simulink library "tqd"  (R2021b)
settings: Solver=VariableStepAuto  StartTime=0.0  StopTime=10.0  RelTol=1e-3
undefined symbols (not defined in the file): ATQD_AfterTqMinGain_X_Deg, ATQD_APSCreepBaseTqD_X_kph, ATQD_APSCreepBaseTqD_Y_Deg, ATQD_APSCreepBaseTqR_X_kph, ATQD_APSCreepBaseTqR_Y_Deg, ATQD_APSCreepIterm_X_kph, ATQD_APSCreepIterm_Y_kph, ATQD_APSCreepPterm_X_kph, ATQD_APSCreepPterm_Y_kph, ATQD_APSDecReq_X_kph, ATQD_APSDecReq_Y_mps2, ATQD_APSDecReqCMD_X_kph, ATQD_APSDecReqTs_X_pct, ATQD_APSDecTimeGain_X_Deg, ATQD_APSDecTimeGain_Y_s, ATQD_APSReqLowSpd_X_Deg, ATQD_AutoHoldReleaseBPS_X_Deg, ATQD_AWDLoadTrqnsGain_X_kg, ATQD_AWDLoadTrqnsGain_Y_pct, ATQD_BOSEnBPSPosn_X_kph, ATQD_BOSMap_X_rpm, ATQD_BOSMap_Y_pct, ATQD_CreepBaseTqD_X_kph, ATQD_CreepBaseTqD_Y_Deg, ATQD_CreepBaseTqR_X_kph, ATQD_CreepBaseTqR_Y_Deg, ATQD_CreepBPSDisPosn_X_Deg, ATQD_CreepBPSDisPosnR_X_Deg, ATQD_CreepBPSEnPosn_X_Deg, ATQD_CreepBPSEnPosnR_X_Deg, ATQD_CreepDeltaTq_X_kph, ATQD_CreepIterm_X_kph, ATQD_CreepIterm_Y_kph, ATQD_CreepItermMaxLimit_X_pct, ATQD_CreepPreloadTime_X_kph, ATQD_CreepPreloadTq_X_kph, ATQD_CreepPreloadTq_Y_s, ATQD_CreepProtTq_X_Deg, ATQD_CreepPterm_X_kph, ATQD_CreepPterm_Y_kph, ATQD_CreepRrTqSpRat_X_rpm, ATQD_CreepRrTqSpRat_Y_Nm, ATQD_CreepTargetSpdD_X_pct, ATQD_CreepTargetSpdR_X_pct, ATQD_ECOTqMapD_X_rpm, ATQD_ECOTqMapD_Y_pct, ATQD_EMTqMapD_X_rpm, ATQD_EMTqMapD_Y_pct, ATQD_EOPDTqMapDCon_X_rpm, ATQD_EOPDTqMapDCon_Y_Deg, ATQD_EscapeModePedTq_X_pct, ATQD_EscapeModePedTq_Y_rpm, ATQD_EscapeModePedTqFr_X_pct, ATQD_EscapeModePedTqFr_Y_rpm, ATQD_EstInitVehWeight_X_c, ATQD_FAfterTqCMDGain_X_rpm, ATQD_FAfterTqCMDGain_Y_pct, ATQD_FrLossMAPLowV_X_rpm, ATQD_FrLossMAPLowV_Y_Nm, ATQD_FrMotActReduce_X_rpm ... (+772)
libraries: simulink x211, hcu_lib x179, tqr x3
(part 11 of 28)

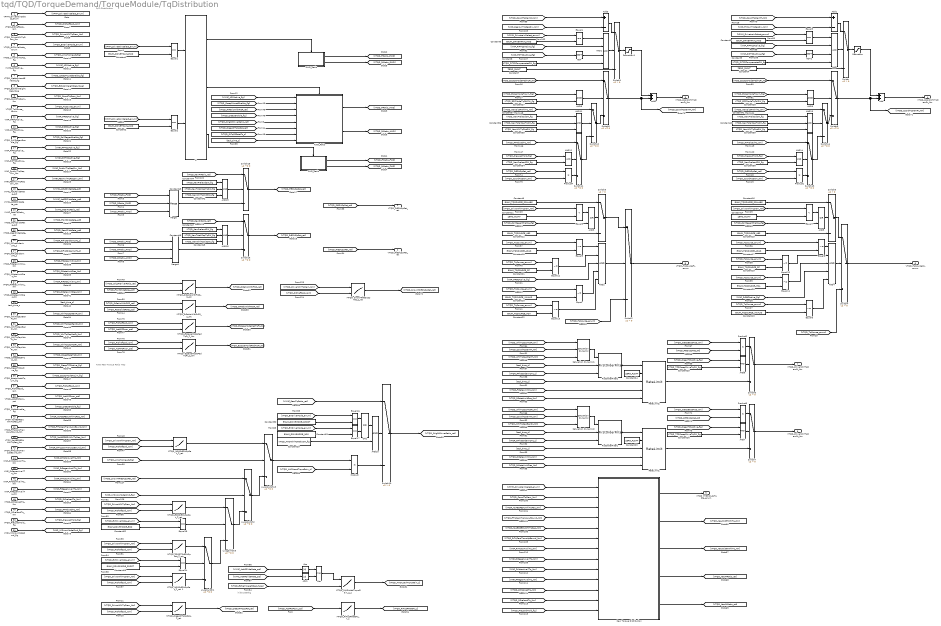
== system tqd/TQD/TorqueDemand/TorqueModule/TqDistribution ==
  note: AWD Rear Torque Ratio Map
  note: Fr/Rr Distribution
  note: initia:2000kg
  VPMM_DrivetrainSelect_enum : Inport
  VTQD_RrShaftSpd_rpm : Inport  Port=2
  VTQD_DriverWhlTqDem_Nm : Inport  Port=3
  VTQD_EVDriveMode_enum : Inport  Port=4
  VTQD_LimpHomeAct_flg : Inport  Port=5
  VVMC_APSActive_flg : Inport  Port=6
  VTQD_CreepPrLoadEnable_flg : Inport  Port=7
  VTQD_EstVehWeightResult_kg : Inport  Port=8
  VTQD_CoordTqDem_Nm : Inport  Port=9
  VTQD_TqSource_enum : Inport  Port=10
  VINP_FrRBCActive_flg : Inport  Port=11
  VINP_RrRBCActive_flg : Inport  Port=12
  VTQD_RollRegenEnable_flg : Inport  Port=13
  VINP_FrPTCSActive_flg : Inport  Port=14
  VINP_RrPTCSActive_flg : Inport  Port=15
  VINP_FrntAxlTrqReqDrv_Nm : Inport  Port=16
  VINP_RearAxlTrqReqDrv_Nm : Inport  Port=17
  VVMC_ActLRSlideRate_pct : Inport  Port=18
  VVMC_ActRRSlideRate_pct : Inport  Port=19
  VVMC_RearTqRatio_rat : Inport  Port=20
  VTQD_FrontSlideRate_pct : Inport  Port=21
  VTQD_RearSlideRate_pct : Inport  Port=22
  VTQR_FrFirstOrderInpTs_c : Inport  Port=23
  VTQR_RrFirstOrderInpTs_c : Inport  Port=24
  VTQR_FrRateLimitInc_Nm : Inport  Port=25
  VTQR_FrRateLimitDec_Nm : Inport  Port=26
  VTQR_RrRateLimitInc_Nm : Inport  Port=27
  VTQR_RrRateLimitDec_Nm : Inport  Port=28
  task_time_s : Inport  Port=29
  VTQD_WhlTqCapGenFr_Nm : Inport  Port=30
  VTQD_WhlTqCapGenRr_Nm : Inport  Port=31
  VTQD_WhlTqCapMotFr_Nm : Inport  Port=32
  VTQD_WhlTqCapMotRr_Nm : Inport  Port=33
  VTQD_CreepBaseTqD_Nm : Inport  Port=34
  VTQD_CreepTCSActive_flg : Inport  Port=35
  VTQD_EscapModeTqLim_flg : Inport  Port=36
  VTQD_FrShaftSpd_rpm : Inport  Port=37
  VTQD_ActAPSPosn_pct : Inport  Port=38
  VTQD_CreepEnable_flg : Inport  Port=39
  VTQR_NoABSFEDUWhlTqReq_Nm : Inport  Port=40
  VTQR_FrTqZeroTransLowBound_Nm : Inport  Port=41
  VTQR_NoABSREDUWhlTqReq_Nm : Inport  Port=42
  VTQR_RrTqZeroTransUpBound_Nm : Inport  Port=43
  VINP_RrMotorAvailTq_Nm : Inport  Port=44
  VINP_RrRegenAvailTq_Nm : Inport  Port=45
  VINP_FrMotorAvailTq_Nm : Inport  Port=46
  VINP_FrRegenAvailTq_Nm : Inport  Port=47
  VTQD_RrPreloadTq_Nm : Inport  Port=48
  VTQD_FrPreloadTq_Nm : Inport  Port=49
  VTQD_PreLoadHold_flg : Inport  Port=50
  VINP_IVISnowModeCmd_flg : Inport  Port=51
  AND : Logic  Inputs=4  AllPortsSameDT=off  OutDataTypeStr=boolean
  AND1 : Logic  Inputs=4  AllPortsSameDT=off  OutDataTypeStr=boolean
  AND{6..10,12,14} (7 alike) : Logic  AllPortsSameDT=off  OutDataTypeStr=boolean
  AND{11,13,15..16} (4 alike) : Logic  Inputs=3  AllPortsSameDT=off  OutDataTypeStr=boolean
  AND2 : Logic  Inputs=5  AllPortsSameDT=off  OutDataTypeStr=boolean
  AND3 : Logic  Operator=OR  AllPortsSameDT=off  OutDataTypeStr=boolean
  AND4 : Logic  Inputs=5  AllPortsSameDT=off  OutDataTypeStr=boolean
  AND5 : Logic  Operator=OR  AllPortsSameDT=off  OutDataTypeStr=boolean
  AWD_Ratio : Subsystem  TreatAsAtomicUnit=on
  Abs : Abs
  Abs1 : Abs
  Add : Sum
  Add1 : Sum  Inputs=+-
  Add2 : Sum
  Add3 : Sum  Inputs=+-
  Constant1 : Constant  Value=ENUM_DRIVETRAIN_RWD  VectorParams1D=off  SampleTime=-1
  Constant10 : Constant  Value=ENUM_TQSOURCE_INVALID  VectorParams1D=off  SampleTime=-1
  Constant{4,7,11,14} (4 alike) : Constant  Value=ZERO_FLOAT  VectorParams1D=off  SampleTime=-1
  Constant12 : Constant  Value=ENUM_TQSOURCE_ABS  VectorParams1D=off  SampleTime=-1
  Constant13 : Constant  Value=ENUM_TQSOURCE_INVALID  VectorParams1D=off  SampleTime=-1
  Constant15 : Constant  Value=ENUM_TQSOURCE_ABS  VectorParams1D=off  SampleTime=-1
  Constant16 : Constant  Value=ENUM_TQSOURCE_ROLLABS  VectorParams1D=off  SampleTime=-1
  Constant17 : Constant  Value=ENUM_TQSOURCE_ADAS  VectorParams1D=off  SampleTime=-1
  Constant18 : Constant  Value=ENUM_TQSOURCE_ADAS  VectorParams1D=off  SampleTime=-1
  Constant19 : Constant  Value=ENUM_TQSOURCE_CC  SampleTime=-1
  Constant2 : Constant  Value=ENUM_DRIVETRAIN_AWD  VectorParams1D=off  SampleTime=-1
  Constant20 : Constant  Value=ENUM_TQSOURCE_MSA  SampleTime=-1
  Constant21 : Constant  Value=ENUM_TQSOURCE_CC  SampleTime=-1
  Constant22 : Constant  Value=ENUM_TQSOURCE_MSA  SampleTime=-1
  Constant23 : Constant  Value=ZERO_FLOAT
  Constant24 : Constant  Value=ZERO_FLOAT
  Constant25 : Constant  Value=KTQD_TCSCreepDriveTqSW_flg  VectorParams1D=off  SampleTime=-1
  Constant26 : Constant  Value=KTQD_TCSCreepDriveTqSW_flg  VectorParams1D=off  SampleTime=-1
  Constant27 : Constant  Value=KTQD_ESCModeTqCtrlSW_flg  VectorParams1D=off  SampleTime=-1
  Constant28 : Constant  Value=KTQD_ESCModeTqCtrlSW_flg  VectorParams1D=off  SampleTime=-1
  Constant29 : Constant  Value=KTQD_AWDWhlTqRatioSW_flg
  Constant3 : Constant  Value=ENUM_DRIVETRAIN_AWD  VectorParams1D=off  SampleTime=-1
  Constant30 : Constant  Value=ENUM_DRIVEMODE_SPORT
  Constant31 : Constant  Value=ENUM_DRIVEMODE_NRM
  Constant32 : Constant  Value=ENUM_DRIVEMODE_ECO
  Constant33 : Constant  Value=ENUM_DRIVEMODE_SPORT
  Constant{34,37..38,41,44,47} (6 alike) : Constant  Value=KTQD_NewPrelaodSW_flg  VectorParams1D=off  SampleTime=-1
  Constant{35,39,42,45} (4 alike) : Constant  Value=KTQD_NewWhlTqDistSW_flg  VectorParams1D=off  SampleTime=-1
  Constant{36,40,43,46} (4 alike) : Constant  Value=KTQD_NewTotalCapTqSW_flg  VectorParams1D=off  SampleTime=-1
  Constant5 : Constant  Value=KTQD_RrTCSCompensateSW_flg  VectorParams1D=off  SampleTime=-1
  Constant6 : Constant  Value=ENUM_DRIVETRAIN_AWD  VectorParams1D=off  SampleTime=-1
  Constant8 : Constant  Value=KTQD_FrTCSCompensateSW_flg  VectorParams1D=off  SampleTime=-1
  Constant9 : Constant  Value=ENUM_TQSOURCE_ROLLABS  VectorParams1D=off  SampleTime=-1
  Equal{,6,8..13} (8 alike) : RelationalOperator  Operator=~=  OutDataTypeStr=boolean  RndMeth=Simplest
  Equal{1..4,14..17} (8 alike) : RelationalOperator  Operator===  OutDataTypeStr=boolean  RndMeth=Simplest
  Equal5 : RelationalOperator  Operator=<  OutDataTypeStr=boolean  RndMeth=Simplest
  Equal7 : RelationalOperator  Operator=<  OutDataTypeStr=boolean  RndMeth=Simplest
  FWD_Ratio : Subsystem  TreatAsAtomicUnit=on
  FirstOrderFilter1 : hcu_lib/Basic_Blocks/FirstOrderFilter
  FirstOrderFilter2 : hcu_lib/Basic_Blocks/FirstOrderFilter
  If : If  NumInputs=2  IfExpression=u1 ~= 0  ElseIfExpressions=u2 ~= 0
  LiuzgSwitch{1..3,13} (4 alike) : Switch  Criteria=u2 ~= 0
      settings: AttributesFormatString=<%<Criteria>>
  MTQD_AWDLoadTrqnsGain_Z_c : Lookup_n-D  BreakpointsForDimension1=ATQD_AWDLoadTrqnsGain_Y_pct  BreakpointsForDimension2=ATQD_AWDLoadTrqnsGain_X_kg  Table=MTQD_AWDLoadTrqnsGain_Z_c  ExtrapMethod=Clip  InternalRulePriority=Speed  RndMeth=Simplest  InputSameDT=on
      settings: InputPortMap=u0,u1
  MTQD_CreepRrTqSpRat_Z_rat : Lookup_n-D  BreakpointsForDimension1=ATQD_CreepRrTqSpRat_Y_Nm  BreakpointsForDimension2=ATQD_CreepRrTqSpRat_X_rpm  Table=MTQD_CreepRrTqSpRat_Z_rat  ExtrapMethod=Clip  InternalRulePriority=Speed  RndMeth=Simplest  InputSameDT=on
      settings: InputPortMap=u0,u1
  MTQD_ECORrEDUSpRat_Z_rat : Lookup_n-D  BreakpointsForDimension1=ATQD_NRMRrEDUSpRat_Y_Nm  BreakpointsForDimension2=ATQD_NRMRrEDUSpRat_X_rpm  Table=MTQD_ECORrEDUSpRat_Z_rat  ExtrapMethod=Clip  InternalRulePriority=Speed  RndMeth=Simplest  InputSameDT=on
      settings: InputPortMap=u0,u1
  MTQD_EscapeModePedTqFr_Z_Nm : Lookup_n-D  BreakpointsForDimension1=ATQD_EscapeModePedTqFr_Y_rpm  BreakpointsForDimension2=ATQD_EscapeModePedTqFr_X_pct  Table=MTQD_EscapeModePedTqFr_Z_Nm  InternalRulePriority=Speed  RndMeth=Simplest  InputSameDT=on
      settings: InputPortMap=u0,u1
  MTQD_EscapeModePedTqRr_Z_Nm : Lookup_n-D  BreakpointsForDimension1=ATQD_EscapeModePedTqFr_Y_rpm  BreakpointsForDimension2=ATQD_EscapeModePedTqFr_X_pct  Table=MTQD_EscapeModePedTqRr_Z_Nm  InternalRulePriority=Speed  RndMeth=Simplest  InputSameDT=on
      settings: InputPortMap=u0,u1
  "MTQD_NRMRrEDUSpRat_Z_rat  " : Lookup_n-D  BreakpointsForDimension1=ATQD_NRMRrEDUSpRat_Y_Nm  BreakpointsForDimension2=ATQD_NRMRrEDUSpRat_X_rpm  Table=MTQD_NRMRrEDUSpRat_Z_rat  ExtrapMethod=Clip  InternalRulePriority=Speed  RndMeth=Simplest  InputSameDT=on
      settings: InputPortMap=u0,u1
  MTQD_NRMRrEDUSpRat_Z_rat  1 : Lookup_n-D  BreakpointsForDimension1=ATQD_NRMRrEDUSpRat_Y_Nm  BreakpointsForDimension2=ATQD_NRMRrEDUSpRat_X_rpm  Table=MTQD_NRMRrEDUSpRat_Z_rat  ExtrapMethod=Clip  InternalRulePriority=Speed  RndMeth=Simplest  InputSameDT=on
      settings: InputPortMap=u0,u1
  MTQD_RrRatioWithFrSR_Z_rat : Lookup_n-D  BreakpointsForDimension1=ATQD_RrRatioWithFrSR_Y_rat  BreakpointsForDimension2=ATQD_RrRatioWithFrSR_X_pct  Table=MTQD_RrRatioWithFrSR_Z_rat  ExtrapMethod=Clip  UseLastTableValue=on  InternalRulePriority=Speed  RndMeth=Simplest  InputSameDT=on
      settings: InputPortMap=u0,u1
  MTQD_RrRatioWithRrSR_Z_rat : Lookup_n-D  BreakpointsForDimension1=ATQD_RrRatioWithFrSR_Y_rat  BreakpointsForDimension2=ATQD_RrRatioWithFrSR_X_pct  Table=MTQD_RrRatioWithRrSR_Z_rat  ExtrapMethod=Clip  UseLastTableValue=on  InternalRulePriority=Speed  RndMeth=Simplest  InputSameDT=on
      settings: InputPortMap=u0,u1
  MTQD_RrTqSRRateTs_Y_c : Lookup_n-D  NumberOfTableDimensions=1  BreakpointsForDimension1=ATQD_RrTqSRRateTs_X_pct  Table=MTQD_RrTqSRRateTs_Y_c  InternalRulePriority=Speed  RndMeth=Simplest  InputSameDT=on
  "MTQD_SPORTRrEDUSpRat_Z_rat " : Lookup_n-D  BreakpointsForDimension1=ATQD_NRMRrEDUSpRat_Y_Nm  BreakpointsForDimension2=ATQD_NRMRrEDUSpRat_X_rpm  Table=MTQD_SPORTRrEDUSpRat_Z_rat  ExtrapMethod=Clip  InternalRulePriority=Speed  RndMeth=Simplest  InputSameDT=on
      settings: InputPortMap=u0,u1
  MTQD_SnowMRrEDUSpRat_Z_rat : Lookup_n-D  BreakpointsForDimension1=ATQD_NRMRrEDUSpRat_Y_Nm  BreakpointsForDimension2=ATQD_NRMRrEDUSpRat_X_rpm  Table=MTQD_SnowMRrEDUSpRat_Z_rat  ExtrapMethod=Clip  InternalRulePriority=Speed  RndMeth=Simplest  InputSameDT=on
      settings: InputPortMap=u0,u1
  Max : MinMax  Function=max  Inputs=2
  Merge : Merge  Inputs=3
  Merge1 : Merge  Inputs=3
  NOT : Logic  Operator=NOT  AllPortsSameDT=off  OutDataTypeStr=boolean
  NOT2 : Logic  Operator=NOT  AllPortsSameDT=off  OutDataTypeStr=boolean
  New Torque Distribution : Subsystem
  OR2 : Logic  Operator=OR  AllPortsSameDT=off  OutDataTypeStr=boolean
  Product{,1..4} (5 alike) : Product
  RWD_Ratio : Subsystem  TreatAsAtomicUnit=on
  RateLimit1 : tqr/TQR/Determine Torque Request/TorqueArbitrament/TorqueSmooth/RateLimit
  RateLimit2 : tqr/TQR/Determine Torque Request/TorqueArbitrament/TorqueSmooth/RateLimit
  Saturation : Saturate  UpperLimit=KTQD_TCSCompUpLimit_Nm  LowerLimit=ZERO_FLOAT
  Saturation Dynamic1 : simulink/Discontinuities/Saturation Dynamic  OutMin=[]  OutMax=[]  OutDataTypeStr=Inherit: Same as second input  OutDataType=fixdt(1, 16)  OutScaling=2^-10  DoSatur=off
  Saturation Dynamic2 : simulink/Discontinuities/Saturation Dynamic  OutMin=[]  OutMax=[]  OutDataTypeStr=Inherit: Same as second input  OutDataType=fixdt(1, 16)  OutScaling=2^-10  DoSatur=off
  Saturation1 : Saturate  UpperLimit=KTQD_TCSCompUpLimit_Nm  LowerLimit=ZERO_FLOAT
  Switch{,1..7,10} (9 alike) : Switch  Criteria=u2 > Threshold
  Switch{8..9,11..16} (8 alike) : Switch  Criteria=u2 ~= 0
      settings: AttributesFormatString=%<Criteria>
  VTQD_FrEDUSpRat_rat : Outport
  VTQD_RrEDUSpRat_rat : Outport  Port=2
  VTQD_CoordWhlTqDemFr_Nm : Outport  Port=3
  VTQD_CoordWhlTqDemRr_Nm : Outport  Port=4
  VTQD_TqSourceFr_enum : Outport  Port=5
  VTQD_TqSourceRr_enum : Outport  Port=6
  VTQD_DriverWhlTqDemFr_Nm : Outport  Port=7
  VTQD_DriverWhlTqDemRr_Nm : Outport  Port=8
  VTQD_TMEnOutpTqSta_enum : Outport  Port=9
  wires:
  VPMM_DrivetrainSelect_enum/1 -> [VPMM_DrivetrainSelect_enum]
  Constant1/1 -> Equal1/2
  [VPMM_DrivetrainSelect_enum] -> Equal1/1
  [VPMM_DrivetrainSelect_enum] -> Equal2/1
  Constant2/1 -> Equal2/2
  Equal2/1 -> If/2
  FWD_Ratio/1(VTQD_FrRatio_FWD) -> [VTQD_FrRatio_FWD]  "VTQD_FrRatio_FWD"
  FWD_Ratio/2(VTQD_RrRatio_FWD) -> [VTQD_RrRatio_FWD]  "VTQD_RrRatio_FWD"
  RWD_Ratio/1(VTQD_FrRatio_RWD) -> [VTQD_FrRatio_RWD]  "VTQD_FrRatio_RWD"
  RWD_Ratio/2(VTQD_RrRatio_RWD) -> [VTQD_RrRatio_RWD]  "VTQD_RrRatio_RWD"
  [VTQD_FrRatio_FWD] -> Merge/1
  [VTQD_FrRatio_RWD] -> Merge/2
  [VTQD_FrRatio_AWD] -> Merge/3
  [VTQD_RrRatio_FWD] -> Merge1/1
  [VTQD_RrRatio_RWD] -> Merge1/2
  [VTQD_RrRatio_AWD] -> Merge1/3
  AWD_Ratio/1(VTQD_FrRatio_AWD) -> [VTQD_FrRatio_AWD]  "VTQD_FrRatio_AWD"
  AWD_Ratio/2(VTQD_RrRatio_AWD) -> [VTQD_RrRatio_AWD]  "VTQD_RrRatio_AWD"
  Equal1/1 -> If/1
  If/1 -> RWD_Ratio/Action
  If/2 -> AWD_Ratio/Action
  If/3 -> FWD_Ratio/Action
  VTQD_RrShaftSpd_rpm/1 -> [VTQD_RrShaftSpd_rpm]
  VTQD_DriverWhlTqDem_Nm/1 -> [VTQD_DriverWhlTqDem_Nm]
  VTQD_EVDriveMode_enum/1 -> [VTQD_EVDriveMode_enum]
  VTQD_LimpHomeAct_flg/1 -> [VTQD_LimpHomeAct_flg]
  VTQD_CreepPrLoadEnable_flg/1 -> [VTQD_CreepPrLoadEnable_flg]
  [VTQD_CreepPrLoadEnable_flg] -> AWD_Ratio/2(VTQD_CreepPrLoadEnable_flg)
  [VVMC_APSActive_flg] -> AWD_Ratio/1(VVMC_APSActive_flg)
  VVMC_APSActive_flg/1 -> [VVMC_APSActive_flg]
  VTQD_EstVehWeightResult_kg/1 -> [VTQD_EstVehWeightResult_kg]
  [VTQD_FrEDUSpRat_rat] -> VTQD_FrEDUSpRat_rat/1
  [VTQD_RrEDUSpRat_rat] -> VTQD_RrEDUSpRat_rat/1
  Switch3/1 -> Switch2/1
  AND4/1 -> Switch4/2
  Add2/1 -> VTQD_CoordWhlTqDemFr_Nm/1  "VTQD_CoordWhlTqDemFr_Nm"
  Equal5/1 -> AND3/1
  [VINP_FrPTCSActive_flg] -> AND/2
  Equal7/1 -> AND5/1
  [VTQD_DriverWhlTqDem_Nm] -> Equal5/1
  [VTQD_TqSource_enum] -> Switch4/3
  [VTQD_RollRegenEnable_flg] -> AND5/2
  [VTQD_RollRegenEnable_flg] -> AND3/2
  Constant6/1 -> Equal4/2
  Constant12/1 -> Switch3/3
  Switch5/1 -> Switch4/1
  Constant9/1 -> Switch3/1
  AND/1 -> Switch/2
  AND1/1 -> Switch1/2
  [VTQD_DriverWhlTqDem_Nm] -> Equal7/1
  Constant14/1 -> Equal7/2
  AND5/1 -> Switch5/2
  Constant10/1 -> Equal/2
  [VINP_RearAxlTrqReqDrv_Nm] -> Add3/2
  Constant16/1 -> Switch5/1
  Constant4/1 -> Switch/3
  Switch4/1 -> VTQD_TqSourceRr_enum/1  "VTQD_TqSourceRr_enum"
  Constant11/1 -> Equal5/2
  [VINP_RrPTCSActive_flg] -> NOT2/1
  AND3/1 -> Switch3/2
  [VINP_FrntAxlTrqReqDrv_Nm] -> Add1/2
  [VTQD_TqSource_enum] -> Switch2/3
  [VTQD_RrEDUSpRat_rat] -> Product1/1
  [VTQD_TqSource_enum] -> Equal6/1
  [VPMM_DrivetrainSelect_enum] -> Equal4/1
  [VTQD_CoordTqDem_Nm] -> Product1/2
  Constant5/1 -> AND/4
  Constant13/1 -> Equal6/2
  NOT/1 -> AND1/3
  Add/1 -> VTQD_CoordWhlTqDemRr_Nm/1  "VTQD_CoordWhlTqDemRr_Nm"
  Equal4/1 -> AND1/1
  [VPMM_DrivetrainSelect_enum] -> Equal3/1
  [VINP_FrPTCSActive_flg] -> NOT/1
  [VTQD_CoordTqDemRr_Nm] -> Add3/1
  Equal3/1 -> AND/1
  [VTQD_TqSource_enum] -> Equal/1
  Constant3/1 -> Equal3/2
  Constant8/1 -> AND1/4
  Switch/1 -> Saturation/1
  Add3/1 -> Switch1/1
  Switch1/1 -> Saturation1/1
  Add1/1 -> Switch/1
  Constant7/1 -> Switch1/3
  Constant15/1 -> Switch5/3
  Saturation1/1 -> Add2/1  "VTQD_FrTCSCompensateTq_Nm"
  NOT2/1 -> AND/3
  [VINP_RrPTCSActive_flg] -> AND1/2
  Switch2/1 -> VTQD_TqSourceFr_enum/1  "VTQD_TqSourceFr_enum"
  [VTQD_CoordTqDemFr_Nm] -> Add1/1
  Saturation/1 -> Add/1  "VTQD_RrTCSCompensateTq_Nm"
  VINP_RrPTCSActive_flg/1 -> [VINP_RrPTCSActive_flg]
  VINP_RearAxlTrqReqDrv_Nm/1 -> [VINP_RearAxlTrqReqDrv_Nm]
  VTQD_CoordTqDem_Nm/1 -> [VTQD_CoordTqDem_Nm]
  VINP_FrntAxlTrqReqDrv_Nm/1 -> [VINP_FrntAxlTrqReqDrv_Nm]
  VTQD_RollRegenEnable_flg/1 -> [VTQD_RollRegenEnable_flg]
  VINP_RrRBCActive_flg/1 -> [VINP_RrRBCActive_flg]
  VTQD_TqSource_enum/1 -> [VTQD_TqSource_enum]
  VINP_FrRBCActive_flg/1 -> [VINP_FrRBCActive_flg]
  VINP_FrPTCSActive_flg/1 -> [VINP_FrPTCSActive_flg]
  VVMC_ActLRSlideRate_pct/1 -> [VVMC_ActLRSlideRate_pct]
  VVMC_ActRRSlideRate_pct/1 -> [VVMC_ActRRSlideRate_pct]
  Constant17/1 -> Equal8/2
  [VTQD_TqSource_enum] -> Equal8/1
  Equal6/1 -> AND4/5
  Equal8/1 -> AND4/1
  [VINP_RrRBCActive_flg] -> AND4/4
  AND2/1 -> Switch2/2
  [VINP_FrRBCActive_flg] -> AND2/3
  [VTQD_TqSource_enum] -> Equal9/1
  Constant18/1 -> Equal9/2
  Equal/1 -> AND2/4
  Equal9/1 -> AND2/1
  [VTQD_TqSource_enum] -> Equal10/1
  Constant19/1 -> Equal10/2
  Equal10/1 -> AND4/2
  Constant20/1 -> Equal11/2
  [VTQD_TqSource_enum] -> Equal11/1
  Equal11/1 -> AND4/3
  [VTQD_TqSource_enum] -> Equal13/1
  Constant22/1 -> Equal13/2
  Constant21/1 -> Equal12/2
  [VTQD_TqSource_enum] -> Equal12/1
  Equal12/1 -> AND2/2
  Equal13/1 -> AND2/5
  VVMC_RearTqRatio_rat/1 -> [VVMC_RearTqRatio_rat]
  VTQD_RearSlideRate_pct/1 -> [VTQD_RearSlideRate_pct]
  VTQD_FrontSlideRate_pct/1 -> [VTQD_FrontSlideRate_pct]
  [VTQD_RearSlideRate_pct] -> MTQD_RrRatioWithRrSR_Z_rat/2
  MTQD_RrRatioWithFrSR_Z_rat/1 -> [VTQD_RrRatioWithFrSR_rat]  "VTQD_RrRatioWithFrSR_rat"
  MTQD_RrRatioWithRrSR_Z_rat/1 -> [VTQD_RrRatioWithRrSR_rat]  "VTQD_RrRatioWithRrSR_rat"
  [VTQD_RrRatioWithRrSR_rat] -> AWD_Ratio/3(VTQD_RrRatioWithRrSR_rat)
  [VTQD_CreepEnable_flg] -> AWD_Ratio/4(VTQD_CreepEnable_flg)
  [VTQD_FrontSlideRate_pct] -> MTQD_RrRatioWithFrSR_Z_rat/2
  [VTQD_RrRatioWithFrSR_rat] -> MTQD_RrRatioWithRrSR_Z_rat/1
  task_time_s/1 -> [task_time_s]
  VTQR_FrRateLimitInc_Nm/1 -> [VTQR_FrRateLimitInc_Nm]
  VTQR_RrRateLimitDec_Nm/1 -> [VTQR_RrRateLimitDec_Nm]
  VTQR_FrRateLimitDec_Nm/1 -> [VTQR_FrRateLimitDec_Nm]
  VTQR_FrFirstOrderInpTs_c/1 -> [VTQR_FrFirstOrderInpTs_c]
  VTQR_RrRateLimitInc_Nm/1 -> [VTQR_RrRateLimitInc_Nm]
  VTQR_RrFirstOrderInpTs_c/1 -> [VTQR_RrFirstOrderInpTs_c]
  [VTQR_RrRateLimitInc_Nm] -> RateLimit1/4
  [VTQR_FrRateLimitDec_Nm] -> RateLimit2/5
  [VTQR_RrFirstOrderInpTs_c] -> FirstOrderFilter1/3
  [task_time_s] -> FirstOrderFilter2/2
  [task_time_s] -> RateLimit2/3
  [VTQR_FrRateLimitInc_Nm] -> RateLimit2/4
  [task_time_s] -> FirstOrderFilter1/2
  [VTQR_RrRateLimitDec_Nm] -> RateLimit1/5
  [task_time_s] -> RateLimit1/3
  Constant23/1 -> RateLimit1/2
  Constant24/1 -> RateLimit2/2
  [VTQR_FrFirstOrderInpTs_c] -> FirstOrderFilter2/3
  FirstOrderFilter1/1 -> RateLimit1/1
  FirstOrderFilter2/1 -> RateLimit2/1
  VTQD_WhlTqCapGenRr_Nm/1 -> [VTQD_WhlTqCapGenRr_Nm]
  VTQD_WhlTqCapMotFr_Nm/1 -> [VTQD_WhlTqCapMotFr_Nm]
  VTQD_WhlTqCapMotRr_Nm/1 -> [VTQD_WhlTqCapMotRr_Nm]
  VTQD_WhlTqCapGenFr_Nm/1 -> [VTQD_WhlTqCapGenFr_Nm]
  [VTQD_CoordTqDemFr_Nm] -> Saturation Dynamic1/2
  Saturation Dynamic1/1 -> FirstOrderFilter2/1
  [VTQD_WhlTqCapMotFr_Nm] -> Saturation Dynamic1/1
  [VTQD_WhlTqCapGenFr_Nm] -> Saturation Dynamic1/3
  Saturation Dynamic2/1 -> FirstOrderFilter1/1
  [VTQD_CoordTqDemRr_Nm] -> Saturation Dynamic2/2
  [VTQD_WhlTqCapGenRr_Nm] -> Saturation Dynamic2/3
  [VTQD_WhlTqCapMotRr_Nm] -> Saturation Dynamic2/1
  VTQD_CreepBaseTqD_Nm/1 -> [VTQD_CreepBaseTqD_Nm]
  RateLimit2/1 -> Switch6/3
  Switch6/1 -> VTQD_DriverWhlTqDemFr_Nm/1  "VTQD_DriverWhlTqDemFr_Nm"
  AND6/1 -> Switch6/2
  Product2/1 -> Switch6/1
  [VTQD_CreepBaseTqD_Nm] -> Product2/1
  [VTQD_FrEDUSpRat_rat] -> Product2/2
  VTQD_CreepTCSActive_flg/1 -> [VTQD_CreepTCSActive_flg]
  [VTQD_CreepTCSActive_flg] -> AND6/1
  Constant25/1 -> AND6/2
  [VTQD_CreepTCSActive_flg] -> AND7/1
  Constant26/1 -> AND7/2
  RateLimit1/1 -> Switch7/3
  AND7/1 -> Switch7/2
  [VTQD_CreepBaseTqD_Nm] -> Product3/1
  [VTQD_RrEDUSpRat_rat] -> Product3/2
  Product3/1 -> Switch7/1
  Switch7/1 -> VTQD_DriverWhlTqDemRr_Nm/1  "VTQD_DriverWhlTqDemRr_Nm"
  VTQD_EscapModeTqLim_flg/1 -> [VTQD_EscapModeTqLim_flg]
  [VTQD_FrShaftSpd_rpm] -> MTQD_EscapeModePedTqFr_Z_Nm/1
  [VTQD_RrShaftSpd_rpm] -> MTQD_EscapeModePedTqRr_Z_Nm/1
  VTQD_FrShaftSpd_rpm/1 -> [VTQD_FrShaftSpd_rpm]
  [VTQD_ActAPSPosn_pct] -> MTQD_EscapeModePedTqFr_Z_Nm/2
  [VTQD_ActAPSPosn_pct] -> MTQD_EscapeModePedTqRr_Z_Nm/2
  VTQD_ActAPSPosn_pct/1 -> [VTQD_ActAPSPosn_pct]
  MTQD_EscapeModePedTqFr_Z_Nm/1 -> [VTQD_EscapeModePedTqFr_Nm]  "VTQD_EscapeModePedTqFr_Nm"
  MTQD_EscapeModePedTqRr_Z_Nm/1 -> [VTQD_EscapeModePedTqRr_Nm]  "VTQD_EscapeModePedTqRr_Nm"
  AND8/1 -> Switch8/2
  Switch8/1 -> [VTQD_CoordTqDemFr_Nm], Add2/2  "VTQD_CoordTqDemFr_Nm"
  [VTQD_FrEDUSpRat_rat] -> Product4/1
  [VTQD_CoordTqDem_Nm] -> Product4/2
  [VTQD_EscapeModePedTqFr_Nm] -> Switch8/1
  [VTQD_EscapModeTqLim_flg] -> AND8/1
  Constant27/1 -> AND8/2
  AND9/1 -> Switch9/2
  Constant28/1 -> AND9/2
  [VTQD_EscapModeTqLim_flg] -> AND9/1
  [VTQD_EscapeModePedTqRr_Nm] -> Switch9/1
  Switch9/1 -> [VTQD_CoordTqDemRr_Nm], Add/2  "VTQD_CoordTqDemRr_Nm"
  VTQD_CreepEnable_flg/1 -> [VTQD_CreepEnable_flg]
  [VTQD_OrigRrDriverRatio_rat] -> MTQD_RrRatioWithFrSR_Z_rat/1
  [VTQD_DriverWhlTqDem_Nm] -> "MTQD_NRMRrEDUSpRat_Z_rat  "/1
  Max/1 -> MTQD_AWDLoadTrqnsGain_Z_c/1  "VTQD_AWDLoadTrqnsGain_pct"
  [VTQD_EVDriveMode_enum] -> Equal17/1
  Constant29/1 -> AND10/2
  [VTQD_EVDriveMode_enum] -> Equal15/1
  Constant30/1 -> Equal16/2
  Equal17/1 -> OR2/2
  Switch10/1 -> [VTQD_OrigRrDriverRatio_rat]  "VTQD_OrigRrDriverRatio_rat"
  [VTQD_EVDriveMode_enum] -> Equal16/1
  [VVMC_RearTqRatio_rat] -> Switch10/1
  [VTQD_DriverWhlTqDem_Nm] -> "MTQD_SPORTRrEDUSpRat_Z_rat "/1
  [VVMC_ActLRSlideRate_pct] -> Abs/1
  [VTQD_LimpHomeAct_flg] -> LiuzgSwitch13/2
  OR2/1 -> AND10/1
  Abs1/1 -> Max/2
  Equal14/1 -> LiuzgSwitch1/2
  [VTQD_EVDriveMode_enum] -> Equal14/1
  MTQD_AWDLoadTrqnsGain_Z_c/1 -> [VTQD_AWDLoadTrqnsGain_c]  "VTQD_AWDLoadTrqnsGain_c"
  Abs/1 -> Max/1
  Equal15/1 -> LiuzgSwitch3/2
  Product/1 -> Switch10/3
  Constant33/1 -> Equal14/2
  [VTQD_RrShaftSpd_rpm] -> "MTQD_NRMRrEDUSpRat_Z_rat  "/2
  [VTQD_AWDLoadTrqnsGain_c] -> Product/2
  [VTQD_DriverWhlTqDem_Nm] -> MTQD_ECORrEDUSpRat_Z_rat/1
  "MTQD_SPORTRrEDUSpRat_Z_rat "/1 -> LiuzgSwitch1/1
  [VVMC_ActRRSlideRate_pct] -> Abs1/1
  [VTQD_RrShaftSpd_rpm] -> "MTQD_SPORTRrEDUSpRat_Z_rat "/2
  Constant31/1 -> Equal17/2
  [VTQD_EstVehWeightResult_kg] -> MTQD_AWDLoadTrqnsGain_Z_c/2
  MTQD_ECORrEDUSpRat_Z_rat/1 -> LiuzgSwitch3/1
  Constant32/1 -> Equal15/2
  Equal16/1 -> OR2/1
  [VTQD_RrShaftSpd_rpm] -> MTQD_ECORrEDUSpRat_Z_rat/2
  LiuzgSwitch1/1 -> LiuzgSwitch3/3
  AND10/1 -> Switch10/2
  "MTQD_NRMRrEDUSpRat_Z_rat  "/1 -> LiuzgSwitch13/1
  [VTQD_RrShaftSpd_rpm] -> MTQD_NRMRrEDUSpRat_Z_rat  1/2
  [VTQD_DriverWhlTqDem_Nm] -> MTQD_NRMRrEDUSpRat_Z_rat  1/1
  MTQD_NRMRrEDUSpRat_Z_rat  1/1 -> LiuzgSwitch1/3
  LiuzgSwitch13/1 -> Product/1
  [VTQD_OrigRrDriverRatio_rat] -> AWD_Ratio/5(VTQD_OrigRrDriverRatio_rat)
  [VTQD_DriverWhlTqDem_Nm] -> MTQD_CreepRrTqSpRat_Z_rat/1
  [VTQD_RrShaftSpd_rpm] -> MTQD_CreepRrTqSpRat_Z_rat/2
  MTQD_CreepRrTqSpRat_Z_rat/1 -> [VTQD_CreepRrTqSpRat_rat]  "VTQD_CreepRrTqSpRat_rat"
  [VTQD_CreepRrTqSpRat_rat] -> AWD_Ratio/6(VTQD_CreepRrTqSpRat_rat)
  [VTQD_ActAPSPosn_pct] -> MTQD_RrTqSRRateTs_Y_c/1
  MTQD_RrTqSRRateTs_Y_c/1 -> [VTQD_RrTqSRRateTs_c]  "VTQD_RrTqSRRateTs_c"
  [VTQD_RrTqSRRateTs_c] -> AWD_Ratio/7(VTQD_RrTqSRRateTs_c)
  [task_time_s] -> AWD_Ratio/8(task_time_s)
  [VPMM_DrivetrainSelect_enum] -> New Torque Distribution/1(VPMM_DrivetrainSelect_enum)
  [VTQD_CoordTqDem_Nm] -> New Torque Distribution/2(VTQD_CoordTqDem_Nm)
  [VTQR_NoABSFEDUWhlTqReq_Nm] -> New Torque Distribution/3(VTQR_NoABSFEDUWhlTqReq_Nm)
  [VTQR_FrTqZeroTransLowBound_Nm] -> New Torque Distribution/4(VTQR_FrTqZeroTransLowBound_Nm)
  [VTQR_NoABSREDUWhlTqReq_Nm] -> New Torque Distribution/5(VTQR_NoABSREDUWhlTqReq_Nm)
  [VTQR_RrTqZeroTransUpBound_Nm] -> New Torque Distribution/6(VTQR_RrTqZeroTransUpBound_Nm)
  [VINP_RrMotorAvailTq_Nm] -> New Torque Distribution/7(VINP_RrMotorAvailTq_Nm)
  [VINP_RrRegenAvailTq_Nm] -> New Torque Distribution/8(VINP_RrRegenAvailTq_Nm)
  [VINP_FrMotorAvailTq_Nm] -> New Torque Distribution/9(VINP_FrMotorAvailTq_Nm)
  [VINP_FrRegenAvailTq_Nm] -> New Torque Distribution/10(VINP_FrRegenAvailTq_Nm)
  [VTQD_RrPreloadTq_Nm] -> New Torque Distribution/11(VTQD_RrPreloadTq_Nm)
  [VTQD_FrPreloadTq_Nm] -> New Torque Distribution/12(VTQD_FrPreloadTq_Nm)
  [VTQD_PreLoadHold_flg] -> New Torque Distribution/13(VTQD_PreLoadHold_flg)
  VTQR_NoABSREDUWhlTqReq_Nm/1 -> [VTQR_NoABSREDUWhlTqReq_Nm]
  VTQR_FrTqZeroTransLowBound_Nm/1 -> [VTQR_FrTqZeroTransLowBound_Nm]
  VTQR_NoABSFEDUWhlTqReq_Nm/1 -> [VTQR_NoABSFEDUWhlTqReq_Nm]
  VTQR_RrTqZeroTransUpBound_Nm/1 -> [VTQR_RrTqZeroTransUpBound_Nm]
  VINP_RrMotorAvailTq_Nm/1 -> [VINP_RrMotorAvailTq_Nm]
  VINP_RrRegenAvailTq_Nm/1 -> [VINP_RrRegenAvailTq_Nm]
  VINP_FrMotorAvailTq_Nm/1 -> [VINP_FrMotorAvailTq_Nm]
  VINP_FrRegenAvailTq_Nm/1 -> [VINP_FrRegenAvailTq_Nm]
  VTQD_RrPreloadTq_Nm/1 -> [VTQD_RrPreloadTq_Nm]
  VTQD_FrPreloadTq_Nm/1 -> [VTQD_FrPreloadTq_Nm]
  VTQD_PreLoadHold_flg/1 -> [VTQD_PreLoadHold_flg]
  New Torque Distribution/1(VTQD_TMEnOutpTqSta_enum) -> VTQD_TMEnOutpTqSta_enum/1
  New Torque Distribution/2(VTQD_NewDistFrWhlTq_Nm) -> [VTQD_NewDistFrWhlTq_Nm]
  New Torque Distribution/3(VTQD_NewDistRrWhlTq_Nm) -> [VTQD_NewDistRrWhlTq_Nm]
  New Torque Distribution/4(VTQD_NewFrRatio_rat) -> [VTQD_NewFrRatio_rat]
  New Torque Distribution/5(VTQD_NewRrRatio_rat) -> [VTQD_NewRrRatio_rat]
  [VTQD_FrPreloadTq_Nm] -> Switch11/1
  Product4/1 -> Switch11/3
  Switch11/1 -> Switch12/3
  AND11/1 -> Switch12/2
  AND12/1 -> Switch11/2
  Constant34/1 -> AND12/2
  [VTQD_PreLoadHold_flg] -> AND12/1
  Constant37/1 -> AND11/1
  Constant36/1 -> AND11/2
  Constant35/1 -> AND11/3
  [VTQD_NewDistFrWhlTq_Nm] -> Switch12/1
  Switch12/1 -> Switch8/3
  Constant40/1 -> AND13/2
  Switch13/1 -> Switch14/3
  [VTQD_NewDistRrWhlTq_Nm] -> Switch14/1
  [VTQD_PreLoadHold_flg] -> AND14/1
  AND13/1 -> Switch14/2
  AND14/1 -> Switch13/2
  Constant41/1 -> AND13/1
  [VTQD_RrPreloadTq_Nm] -> Switch13/1
  Constant39/1 -> AND13/3
  Product1/1 -> Switch13/3
  Constant38/1 -> AND14/2
  Switch14/1 -> Switch9/3
  Constant43/1 -> AND15/2
  Constant42/1 -> AND15/3
  Constant44/1 -> AND15/1
  AND15/1 -> Switch15/2
  Merge/1 -> Switch15/3
  Switch15/1 -> [VTQD_FrEDUSpRat_rat]  "VTQD_FrEDUSpRat_rat"
  [VTQD_NewFrRatio_rat] -> Switch15/1
  [VTQD_NewRrRatio_rat] -> Switch16/1
  AND16/1 -> Switch16/2
  Constant45/1 -> AND16/3
  Constant47/1 -> AND16/1
  Constant46/1 -> AND16/2
  Merge1/1 -> Switch16/3
  Switch16/1 -> [VTQD_RrEDUSpRat_rat]  "VTQD_RrEDUSpRat_rat"
  [VTQD_RrShaftSpd_rpm] -> MTQD_SnowMRrEDUSpRat_Z_rat/2
  [VTQD_DriverWhlTqDem_Nm] -> MTQD_SnowMRrEDUSpRat_Z_rat/1
  MTQD_SnowMRrEDUSpRat_Z_rat/1 -> [VTQD_SnowMRrEDUSpRat_rat]  "VTQD_SnowMRrEDUSpRat_rat"
  LiuzgSwitch3/1 -> LiuzgSwitch2/3
  VINP_IVISnowModeCmd_flg/1 -> [VINP_IVISnowModeCmd_flg]
  [VINP_IVISnowModeCmd_flg] -> LiuzgSwitch2/2
  [VTQD_SnowMRrEDUSpRat_rat] -> LiuzgSwitch2/1
  LiuzgSwitch2/1 -> LiuzgSwitch13/3

== system tqd/TQD/TorqueDemand/ShiftModule/GearShiftPosn/Drive Protection ==
  VTQD_ShifterHandleCmd_enum : Inport
  VTQD_GearActualPosn_enum : Inport  Port=2
  VTQD_VehActSpd_kph : Inport  Port=3
  VTQD_AfterAvailableTqDemFr_Nm : Inport  Port=4
  VTQR_NoABSREDUWhlTqReq_Nm : Inport  Port=5
  VTQR_NoABSFEDUWhlTqReq_Nm : Inport  Port=6
  VTQD_AfterAvailableTqDemRr_Nm : Inport  Port=7
  task_time_s : Inport  Port=8
  VTQD_BrkSwSta_flg : Inport  Port=9
  AND : Logic  Inputs=6  AllPortsSameDT=off  OutDataTypeStr=boolean
  AND1 : Logic  Commented=on  AllPortsSameDT=off  OutDataTypeStr=boolean
  AND2 : Logic  Inputs=3  AllPortsSameDT=off  OutDataTypeStr=boolean
  AND3 : Logic  Commented=on  Inputs=3  AllPortsSameDT=off  OutDataTypeStr=boolean
  AND4 : Logic  AllPortsSameDT=off  OutDataTypeStr=boolean
  Abs{,1,3..4} (4 alike) : Abs
  Add : Sum  Commented=on
  Add3 : Sum  Commented=on  Inputs=+++
  Constant1 : Constant  Commented=on  Value=ENUM_SHIFTCOMMAND_N
  Constant{3,6..7,10} (4 alike) : Constant  Value=KTQD_DrivProtEnToNTq_Nm
  Constant11 : Constant  Commented=on  Value=KTQD_CreepDisableSpdofst_kph
  Constant12 : Constant  Value=ENUM_SHIFTCOMMAND_N
  Constant13 : Constant  Value=KTQD_DriveProtVehSpdGain_kph
  Constant14 : Constant  Value=KTQD_DriveProtVehSpdGain_kph
  Constant16 : Constant  Value=KTQD_DrivProtEnSW_flg
  Constant17 : Constant  Value=KTQD_DriveProtDetTime_s
  Constant2 : Constant  Commented=on  Value=KTQD_DriveProtVehSpdGain_kph
  Constant20 : Constant  Commented=on  Value=ZERO_INT
  Constant21 : Constant  Commented=on  Value=ENUM_SHIFTCOMMAND_N
  Constant22 : Constant  Commented=on  Value=ENUM_SHIFTCOMMAND_N
  Constant23 : Constant  Commented=on  Value=ONE_INT
  Constant24 : Constant  Commented=on  Value=ZERO_INT
  Constant25 : Constant  Commented=on  Value=ENUM_SHIFTCOMMAND_NONE
  Constant26 : Constant  Commented=on  Value=KTQD_DriceProtDetTime_s
  Constant27 : Constant  Commented=on  Value=ENUM_SHIFTCOMMAND_D
  Constant29 : Constant  Commented=on  Value=ONE_INT
  Constant4 : Constant  Value=ENUM_GEARACTUALPOSN_D
  Constant5 : Constant  Commented=on  Value=ENUM_SHIFTCOMMAND_NONE
  Constant8 : Constant  Commented=on  Value=KTQD_DriveProtUpCount_c
  Constant9 : Constant  Commented=on  Value=KTQD_CreepEnableSpd_kph
  Delay : Delay  Commented=on  DelayLength=1
  Delay1 : Delay  Commented=on  DelayLength=1
  Delay2 : Delay  Commented=on  DelayLength=1
  Delay{4..8} (5 alike) : Delay  DelayLength=1
  DelayEnable : hcu_lib/Basic_Blocks/DelayEnable
  Detect Increase1 : simulink/Logic and Bit Operations/Detect Increase  Commented=on  vinit=0.0  OutDataTypeStr=boolean
  Equal{,2,6..7} (4 alike) : RelationalOperator  Operator=<=  OutDataTypeStr=boolean  RndMeth=Simplest
  Equal{1,4,12,15..16} (5 alike) : RelationalOperator  Commented=on  Operator===  OutDataTypeStr=boolean  RndMeth=Simplest
  Equal13 : RelationalOperator  Commented=on  Operator=~=  OutDataTypeStr=boolean  RndMeth=Simplest
  Equal14 : RelationalOperator  Commented=on  Operator=~=  OutDataTypeStr=boolean  RndMeth=Simplest
  Equal3 : RelationalOperator  Operator===  OutDataTypeStr=boolean  RndMeth=Simplest
  Equal5 : RelationalOperator  Commented=on  Operator=~=  OutDataTypeStr=boolean  RndMeth=Simplest
  Equal8 : RelationalOperator  Operator===  OutDataTypeStr=boolean  RndMeth=Simplest
  From1 : From  Commented=on  GotoTag=VINP_VehSpeed_kph
  From11 : From  Commented=on  GotoTag=VTQD_DriveProtCount_c
  From13 : From  Commented=on  GotoTag=VTQD_DriveProtDetFinish_flg
  From2 : From  Commented=on  GotoTag=VTQD_GearActualPosn_enum
  From32 : From  Commented=on  GotoTag=VTQD_DriveProtCount_c
  From{7,33..34,36} (4 alike) : From  Commented=on  GotoTag=VINP_ShifterHandleCmd_enum
  From35 : From  Commented=on  GotoTag=VTQD_DrivePortCountReset_flg
  From37 : From  Commented=on  GotoTag=VTQD_DriveProtDetFinish_flg
  From38 : From  Commented=on  GotoTag=VTQD_DriveProtDetFinish_flg
  From39 : From  Commented=on  GotoTag=task_time_s
  From40 : From  Commented=on  GotoTag=VTQD_GearActualPosn_enum
  Goto15 : Goto  Commented=on  GotoTag=VTQD_DrivePortCountReset_flg
  Goto16 : Goto  Commented=on  GotoTag=VTQD_DriveProtCount_c
  Goto17 : Goto  Commented=on  GotoTag=VTQD_DriveProtDetFinish_flg
  Goto9 : Goto  Commented=on  GotoTag=VTQD_DriveProtRemove_flg
  NOT : Logic  Commented=on  Operator=NOT  AllPortsSameDT=off  OutDataTypeStr=boolean
  NOT1 : Logic  Operator=NOT  AllPortsSameDT=off  OutDataTypeStr=boolean
  OR : Logic  Commented=on  Operator=OR  AllPortsSameDT=off  OutDataTypeStr=boolean
  OR1 : Logic  Operator=OR  AllPortsSameDT=off  OutDataTypeStr=boolean
  OR4 : Logic  Commented=on  Operator=OR  AllPortsSameDT=off  OutDataTypeStr=boolean
  OR5 : Logic  Commented=on  AllPortsSameDT=off  OutDataTypeStr=boolean
  Relational Operator1 : RelationalOperator  Commented=on  Operator=>  OutDataTypeStr=boolean  RndMeth=Simplest
  Relational Operator2 : RelationalOperator  Commented=on  OutDataTypeStr=boolean  RndMeth=Simplest
  Relational Operator3 : RelationalOperator  Operator=>  OutDataTypeStr=boolean  RndMeth=Simplest
  Relational Operator4 : RelationalOperator  Operator=<=  OutDataTypeStr=boolean  RndMeth=Simplest
  SR_Latch1 : hcu_lib/Basic_Blocks/SR_Latch  Commented=on
  SR_Latch2 : hcu_lib/Basic_Blocks/SR_Latch  Commented=on
  Switch10 : Switch  Commented=on  Criteria=u2 > Threshold
  Switch9 : Switch  Commented=on  Criteria=u2 > Threshold
  Timer : hcu_lib/Basic_Blocks/Timer  Commented=on
  VTQD_DriveProtRemove_flg : Outport
  VTQD_DriveProtToPsnN_flg : Outport  Port=2
  VTQD_DriveProtEn_flg : Outport  Port=3
  wires:
  [VTQD_DriveProtRemove_flg] -> AND/1
  Delay8/1 -> Equal3/1
  Abs4/1 -> Equal7/1
  Abs3/1 -> Equal6/1
  [VTQD_GearActualPosn_enum] -> Delay8/1
  Abs1/1 -> Equal2/1
  Abs/1 -> Equal/1
  AND2/1 -> VTQD_DriveProtEn_flg/1, DelayEnable/1  "VTQD_DriveProtEn_flg"
  Constant3/1 -> Equal/2
  Constant10/1 -> Equal2/2
  Constant6/1 -> Equal6/2
  Constant7/1 -> Equal7/2
  DelayEnable/1 -> [VTQD_DriveProtRemove_flg]  "VTQD_DriveProtRemove_flg"
  [task_time_s] -> DelayEnable/3
  Constant17/1 -> DelayEnable/2
  Constant16/1 -> AND2/2
  Equal8/1 -> AND2/1
  [VTQD_VehActSpd_kph] -> Relational Operator3/1
  Constant14/1 -> Relational Operator3/2
  Constant12/1 -> Equal8/2
  [VTQD_ShifterHandleCmd_enum] -> Equal8/1
  AND/1 -> [VTQD_DriveProtToPsnN_flg]  "VTQD_DriveProtToPsnN_flg"
  Delay7/1 -> [VTQD_AfterAvailableTqDemFr_Nm]
  Delay6/1 -> [VTQR_NoABSREDUWhlTqReq_Nm]
  Delay5/1 -> [VTQR_NoABSFEDUWhlTqReq_Nm]
  VTQR_NoABSFEDUWhlTqReq_Nm/1 -> Delay5/1
  Delay4/1 -> [VTQD_AfterAvailableTqDemRr_Nm]
  SR_Latch2/1 -> Goto9/1  "VTQD_DriveProtRemove_flg"
  task_time_s/1 -> [task_time_s]
  Constant2/1 -> Add3/1
  Constant11/1 -> Add3/3
  Add3/1 -> Relational Operator1/2
  Constant9/1 -> Add3/2
  VTQD_AfterAvailableTqDemRr_Nm/1 -> Delay4/1
  Equal7/1 -> AND/6
  [VTQD_AfterAvailableTqDemFr_Nm] -> Abs4/1
  Equal6/1 -> AND/5
  [VTQR_NoABSFEDUWhlTqReq_Nm] -> Abs3/1
  [VTQD_DriveProtToPsnN_flg] -> VTQD_DriveProtToPsnN_flg/1
  VTQR_NoABSREDUWhlTqReq_Nm/1 -> Delay6/1
  VTQD_AfterAvailableTqDemFr_Nm/1 -> Delay7/1
  VTQD_VehActSpd_kph/1 -> [VTQD_VehActSpd_kph]
  VTQD_GearActualPosn_enum/1 -> [VTQD_GearActualPosn_enum]
  VTQD_ShifterHandleCmd_enum/1 -> [VTQD_ShifterHandleCmd_enum]
  OR/1 -> SR_Latch2/2
  Equal5/1 -> OR/2
  Equal1/1 -> OR/1
  Constant5/1 -> Equal5/2
  From7/1 -> Equal5/1
  Constant4/1 -> Equal3/2
  Equal3/1 -> AND/4
  [VTQR_NoABSREDUWhlTqReq_Nm] -> Abs1/1
  Equal2/1 -> AND/3
  Equal/1 -> AND/2
  [VTQD_AfterAvailableTqDemRr_Nm] -> Abs/1
  [VTQD_DriveProtRemove_flg] -> VTQD_DriveProtRemove_flg/1
  Constant1/1 -> Equal1/2
  From2/1 -> Equal1/1
  Relational Operator1/1 -> AND3/3
  From1/1 -> Relational Operator1/1
  From11/1 -> Equal4/1
  From13/1 -> AND1/2
  Constant8/1 -> Equal4/2
  AND1/1 -> SR_Latch2/1  "VTQD_DriveProtEn_flg"
  Equal4/1 -> AND1/1
  Delay2/1 -> SR_Latch1/2
  Equal13/1 -> OR5/1
  Switch9/1 -> Add/1
  Switch10/1 -> Delay/1
  Constant24/1 -> Switch10/1
  From35/1 -> Switch10/2
  Detect Increase1/1 -> Switch9/2  "VTQD_ShiftNRiseDet_flg"
  From36/1 -> Equal12/1
  OR4/1 -> Goto15/1  "VTQD_DrivePortCountReset_flg"
  Equal14/1 -> OR5/2
  Add/1 -> Switch10/3
  From33/1 -> Equal13/1
  Constant29/1 -> Equal16/2
  Constant22/1 -> Equal13/2
  Delay/1 -> Add/2, Goto16/1  "VTQD_DriveProtCount_c"
  Equal15/1 -> AND3/2
  From34/1 -> Equal14/1
  Relational Operator2/1 -> Goto17/1  "VTQD_DriveProtDetFinish_flg"
  Constant20/1 -> Switch9/3
  Timer/1 -> Relational Operator2/1  "VTQD_DriveProtDetTime_s"
  OR5/1 -> OR4/2
  AND3/1 -> SR_Latch1/1  "VTQD_DriveProtTimerEn_flg"
  NOT/1 -> Timer/2
  Constant21/1 -> Equal12/2
  Constant25/1 -> Equal14/2
  From39/1 -> Timer/3
  From32/1 -> Equal16/1
  From37/1 -> Delay1/1
  From40/1 -> Equal15/1
  From38/1 -> Delay2/1
  Delay1/1 -> OR4/1
  SR_Latch1/1 -> Timer/1, NOT/1
  Constant27/1 -> Equal15/2
  Constant23/1 -> Switch9/1
  Equal16/1 -> AND3/1
  Equal12/1 -> Detect Increase1/1
  Constant26/1 -> Timer/4, Relational Operator2/2
  OR1/1 -> AND2/3
  Relational Operator3/1 -> OR1/1
  Constant13/1 -> Relational Operator4/2
  [VTQD_VehActSpd_kph] -> Relational Operator4/1
  Relational Operator4/1 -> AND4/1
  AND4/1 -> OR1/2
  [VTQD_BrkSwSta_flg] -> NOT1/1
  NOT1/1 -> AND4/2
  VTQD_BrkSwSta_flg/1 -> [VTQD_BrkSwSta_flg]

== system tqd/TQD/TorqueDemand/Signal_convert/Regen Level Switch Botton/RegenDOWN ==
  note: IF PRESS BOTH then nothing happen
  note: Long press or Short press
  note: If press time more then Long press's limit then go Long press only. Else go short press only. Else if no press.
  note: IF PRESS BOTH then nothing happen
  task_time_s : Inport
  SWC_RegenUp : Inport  Port=2
  SWC_RegenDOWN : Inport  Port=3
  AND : Logic  AllPortsSameDT=off  OutDataTypeStr=boolean
  AND1 : Logic  AllPortsSameDT=off  OutDataTypeStr=boolean
  AND2 : Logic  AllPortsSameDT=off  OutDataTypeStr=boolean
  Constant{1..2,4,7,10} (5 alike) : Constant  Value=FALSE
  Constant3 : Constant  Value=KTQD_RegShortPLim_s
  Default 3 sec : Constant  Value=KTQD_RegLongPLim_s
  DelayEnable_LONG_PRESS : hcu_lib/Basic_Blocks/DelayEnable
  DelayEnable_SHORT_PRESS : hcu_lib/Basic_Blocks/DelayEnable
  Detect Decrease1 : simulink/Logic and Bit Operations/Detect Decrease  vinit=0.0  OutDataTypeStr=boolean
  Detect Decrease2 : simulink/Logic and Bit Operations/Detect Decrease  vinit=0.0  OutDataTypeStr=boolean
  Detect Increase : simulink/Logic and Bit Operations/Detect Increase  vinit=0.0  OutDataTypeStr=boolean
  NOT : Logic  Operator=NOT  AllPortsSameDT=off  OutDataTypeStr=boolean
  NOT1 : Logic  Operator=NOT  AllPortsSameDT=off  OutDataTypeStr=boolean
  SR_Latch : hcu_lib/Basic_Blocks/SR_Latch
  Switch{1..5} (5 alike) : Switch  Criteria=u2 ~= 0
  SWC_RegenDownShort_flg : Outport
  VTQD_RegenDownLongP_flg : Outport  Port=2
  wires:
  Detect Decrease1/1 -> AND/2
  SR_Latch/1 -> [PRESS_BOTH]
  AND2/1 -> SR_Latch/2
  NOT1/1 -> AND2/2
  NOT/1 -> AND2/1
  [SWC_RegenDOWN] -> NOT1/1
  [SWC_RegenUp] -> NOT/1
  Constant4/1 -> Switch5/1
  [PRESS_BOTH] -> Switch5/2
  [SWC_RegenDOWN] -> Switch5/3
  Switch4/1 -> [Short_press_falling_Edge]
  Detect Decrease2/1 -> Switch4/3
  [PRESS_BOTH] -> Switch4/2
  Constant2/1 -> Switch4/1
  Constant1/1 -> Switch3/1
  AND1/1 -> SR_Latch/1
  [SWC_RegenUp] -> AND1/1
  [SWC_RegenDOWN] -> AND1/2
  [PRESS_BOTH] -> Switch3/2
  SWC_RegenDOWN/1 -> [SWC_RegenDOWN]
  SWC_RegenUp/1 -> [SWC_RegenUp]
  Switch3/1 -> [Long_press]
  Switch2/1 -> SWC_RegenDownShort_flg/1
  AND/1 -> Switch2/2
  Switch5/1 -> DelayEnable_LONG_PRESS/1, DelayEnable_SHORT_PRESS/1
  [Short_press_falling_Edge] -> Switch2/3
  Constant10/1 -> Switch2/1
  [Long_press] -> Detect Increase/1, Detect Decrease1/1
  [Short_press_falling_Edge] -> AND/1
  Switch1/1 -> Switch3/3
  DelayEnable_LONG_PRESS/1 -> Switch1/2, Switch1/1
  Constant7/1 -> Switch1/3
  DelayEnable_SHORT_PRESS/1 -> Detect Decrease2/1
  Constant3/1 -> DelayEnable_SHORT_PRESS/2
  [task_time_s] -> DelayEnable_SHORT_PRESS/3
  Default 3 sec/1 -> DelayEnable_LONG_PRESS/2
  [task_time_s] -> DelayEnable_LONG_PRESS/3
  Detect Increase/1 -> VTQD_RegenDownLongP_flg/1
  task_time_s/1 -> [task_time_s]

== system tqd/TQD/TorqueDemand/Signal_convert/Regen Level Switch Botton/RegenUP ==
  note: IF PRESS BOTH then nothing happen
  note: Long press or Short press
  note: If press time more then Long press's limit then go Long press only. Else go short press only. Else if no press.
  note: IF PRESS BOTH then nothing happen
  task_time_s : Inport
  SWC_RegenUp : Inport  Port=2
  SWC_RegenDOWN : Inport  Port=3
  AND : Logic  AllPortsSameDT=off  OutDataTypeStr=boolean
  AND1 : Logic  AllPortsSameDT=off  OutDataTypeStr=boolean
  AND2 : Logic  AllPortsSameDT=off  OutDataTypeStr=boolean
  Constant{1..2,4,7,10} (5 alike) : Constant  Value=FALSE
  Constant3 : Constant  Value=KTQD_RegShortPLim_s
  Default 3 sec : Constant  Value=KTQD_RegLongPLim_s
  DelayEnable_LONG_PRESS : hcu_lib/Basic_Blocks/DelayEnable
  DelayEnable_SHORT_PRESS : hcu_lib/Basic_Blocks/DelayEnable
  Detect Decrease1 : simulink/Logic and Bit Operations/Detect Decrease  vinit=0.0  OutDataTypeStr=boolean
  Detect Decrease2 : simulink/Logic and Bit Operations/Detect Decrease  vinit=0.0  OutDataTypeStr=boolean
  Detect Increase : simulink/Logic and Bit Operations/Detect Increase  vinit=0.0  OutDataTypeStr=boolean
  NOT : Logic  Operator=NOT  AllPortsSameDT=off  OutDataTypeStr=boolean
  NOT1 : Logic  Operator=NOT  AllPortsSameDT=off  OutDataTypeStr=boolean
  SR_Latch : hcu_lib/Basic_Blocks/SR_Latch
  Switch{1..5} (5 alike) : Switch  Criteria=u2 ~= 0
  SWC_RegenUpShort_flg : Outport
  VTQD_RegenUpLongP_flg : Outport  Port=2
  wires:
  Detect Decrease1/1 -> AND/2
  SR_Latch/1 -> [PRESS_BOTH]
  AND2/1 -> SR_Latch/2
  NOT1/1 -> AND2/2
  NOT/1 -> AND2/1
  [SWC_RegenDOWN] -> NOT1/1
  [SWC_RegenUp] -> NOT/1
  Constant4/1 -> Switch5/1
  [PRESS_BOTH] -> Switch5/2
  [SWC_RegenUp] -> Switch5/3
  Switch4/1 -> [Short_press_falling_Edge]
  Detect Decrease2/1 -> Switch4/3
  [PRESS_BOTH] -> Switch4/2
  Constant2/1 -> Switch4/1
  Constant1/1 -> Switch3/1
  AND1/1 -> SR_Latch/1
  [SWC_RegenUp] -> AND1/1
  [SWC_RegenDOWN] -> AND1/2
  [PRESS_BOTH] -> Switch3/2
  SWC_RegenDOWN/1 -> [SWC_RegenDOWN]
  SWC_RegenUp/1 -> [SWC_RegenUp]
  Switch3/1 -> [Long_press]
  Switch2/1 -> SWC_RegenUpShort_flg/1
  AND/1 -> Switch2/2
  Switch5/1 -> DelayEnable_LONG_PRESS/1, DelayEnable_SHORT_PRESS/1
  [Short_press_falling_Edge] -> Switch2/3
  Constant10/1 -> Switch2/1
  [Long_press] -> Detect Increase/1, Detect Decrease1/1
  [Short_press_falling_Edge] -> AND/1
  Switch1/1 -> Switch3/3
  DelayEnable_LONG_PRESS/1 -> Switch1/2, Switch1/1
  Constant7/1 -> Switch1/3
  DelayEnable_SHORT_PRESS/1 -> Detect Decrease2/1
  Constant3/1 -> DelayEnable_SHORT_PRESS/2
  [task_time_s] -> DelayEnable_SHORT_PRESS/3
  Default 3 sec/1 -> DelayEnable_LONG_PRESS/2
  [task_time_s] -> DelayEnable_LONG_PRESS/3
  Detect Increase/1 -> VTQD_RegenUpLongP_flg/1
  task_time_s/1 -> [task_time_s]

== system tqd/TQD/TorqueDemand/Signal_convert/SWC2_Subsystem/Big Mike Combo ==
  task_time_s : Inport
  VINP_SWC2RegenDown_flg : Inport  Port=2
  VINP_SWC2RegenUp_flg : Inport  Port=3
  VINP_SWC2LScrollUpSta_flg : Inport  Port=4
  VINP_SWC2LScrollDownSta_flg : Inport  Port=5
  VINP_SWC2RScrollUpSta_flg : Inport  Port=6
  VINP_SWCDownSta_flg : Inport  Port=7
  VINP_SWC2LScrollPressSta_flg : Inport  Port=8
  VINP_SWC2LADASSta_flg : Inport  Port=9
  VINP_SWC2LDriveModeSta_flg : Inport  Port=10
  VINP_SWC2RScrollPressSta_flg : Inport  Port=11
  VINP_SWCRightSta_flg : Inport  Port=12
  VINP_SWC2RLeftSta_flg : Inport  Port=13
  VPMM_PowerSta_enum : Inport  Port=14
  VTQD_ShiftGearPosn_enum : Inport  Port=15
  Combo Key Detection : Subsystem
  Mode Coordination : Subsystem
  Operation Condition : Subsystem
  Signal Status Detection : Subsystem
  VTQD_StreetFightMode_flg : Outport
  VTQD_ComboKeyPreEn_flg : Outport  Port=2
  VTQD_ComboKeyEn_flg : Outport  Port=3
  VTQD_EngineeringMode_flg : Outport  Port=4
  VTQD_ManufactureMode_flg : Outport  Port=5
  VTQD_ExhibitionMode_flg : Outport  Port=6
  VTQD_DiagnosisOffMode_flg : Outport  Port=7
  VTQD_SysMode_enum : Outport  Port=8
  wires:
  [VSCP_SysMode_enum] -> VTQD_SysMode_enum/1
  Mode Coordination/1(VSCP_SysMode_enum) -> [VSCP_SysMode_enum]
  [VSCP_DiagnosisOffMode_flg] -> Mode Coordination/5(VSCP_DiagnosisOffMode_flg)
  [VSCP_ExhibitionMode_flg] -> Mode Coordination/4(VSCP_ExhibitionMode_flg)
  [VSCP_ManufactureMode_flg] -> Mode Coordination/3(VSCP_ManufactureMode_flg)
  [VSCP_EngineeringMode_flg] -> Mode Coordination/2(VSCP_EngineeringMode_flg)
  [VSCP_StreetFightMode_flg] -> Mode Coordination/1(VSCP_StreetFightMode_flg)
  [VSCP_DiagnosisOffMode_flg] -> VTQD_DiagnosisOffMode_flg/1
  Combo Key Detection/5(VSCP_DiagnosisOffMode_flg) -> [VSCP_DiagnosisOffMode_flg]
  [VSCP_ExhibitionMode_flg] -> VTQD_ExhibitionMode_flg/1
  Combo Key Detection/4(VSCP_ExhibitionMode_flg) -> [VSCP_ExhibitionMode_flg]
  [VSCP_ManufactureMode_flg] -> VTQD_ManufactureMode_flg/1
  Combo Key Detection/3(VSCP_ManufactureMode_flg) -> [VSCP_ManufactureMode_flg]
  Combo Key Detection/2(VSCP_EngineeringMode_flg) -> [VSCP_EngineeringMode_flg]
  [VSCP_EngineeringMode_flg] -> VTQD_EngineeringMode_flg/1
  [VSCP_StreetFightModeOff_flg] -> Combo Key Detection/6(VSCP_StreetFightModeOff_flg)
  [VSCP_ComboKeyEnter_flg] -> Combo Key Detection/5(VSCP_ComboKeyEnter_flg)
  [VSCP_ComboKey_enum] -> Combo Key Detection/4(VSCP_ComboKey_enum)
  [VSCP_ComboKeyReset_flg] -> Combo Key Detection/3(VSCP_ComboKeyReset_flg)
  [VSCP_ComboKeyEn_flg] -> Combo Key Detection/2(VSCP_ComboKeyEn_flg)
  [TASK_TIME_10_MS] -> Combo Key Detection/1(TASK_TIME_10_MS)
  Combo Key Detection/1(VSCP_StreetFightMode_flg) -> [VSCP_StreetFightMode_flg]
  [VSCP_ComboKeyEn_flg] -> Signal Status Detection/16(VSCP_ComboKeyEn_flg)
  [VINP_SWCLeftSta_flg] -> Signal Status Detection/15(VINP_SWCLeftSta_flg)
  [VINP_SWCmodeSta_flg] -> Signal Status Detection/13(VINP_SWCmodeSta_flg)
  [VSCP_ComboKeyEn_flg] -> VTQD_ComboKeyEn_flg/1
  [VSCP_ComboKeyPreEn_flg] -> VTQD_ComboKeyPreEn_flg/1
  VINP_SWC2RLeftSta_flg/1 -> [VINP_SWCLeftSta_flg]
  VINP_SWC2LDriveModeSta_flg/1 -> [VINP_SWCDistanceSta_flg]
  VINP_SWC2RScrollPressSta_flg/1 -> [VINP_SWCmodeSta_flg]
  VINP_SWCRightSta_flg/1 -> [VINP_SWCRightSta_flg]
  [VINP_SWCRightSta_flg] -> Signal Status Detection/14(VINP_SWCRightSta_flg)
  [VINP_SWCDistanceSta_flg] -> Signal Status Detection/12(VINP_SWCDistanceSta_flg)
  [VSCP_SysMode_enum] -> Signal Status Detection/11(VSCP_SysMode_enum)
  VINP_SWC2LScrollPressSta_flg/1 -> [VINP_SWCCANCELSta_flg]
  VINP_SWCDownSta_flg/1 -> [VINP_SWCDownSta_flg]
  task_time_s/1 -> [TASK_TIME_10_MS]
  VINP_SWC2RScrollUpSta_flg/1 -> [VINP_SWCUpSta_flg]
  VINP_SWC2LScrollUpSta_flg/1 -> [VINP_SWCResUpSta_flg]
  Signal Status Detection/5(VSCP_StreetFightModeOff_flg) -> [VSCP_StreetFightModeOff_flg]
  [VINP_SWCCANCELSta_flg] -> Signal Status Detection/8(VINP_SWCCANCELSta_flg)
  VTQD_ShiftGearPosn_enum/1 -> [VINP_ShiftGearPosn_enum]
  [VINP_SWCACCSta_flg] -> Signal Status Detection/10(VINP_SWCACCSta_flg)
  Signal Status Detection/3(VSCP_ComboKeyReset_flg) -> [VSCP_ComboKeyReset_flg]
  [VINP_ShiftGearPosn_enum] -> Operation Condition/2(VINP_ShiftGearPosn_enum)
  VINP_SWC2LADASSta_flg/1 -> [VINP_SWCACCSta_flg]
  VPMM_PowerSta_enum/1 -> [VINP_PwrSta_enum]
  Operation Condition/2(VSCP_ComboKeyEn_flg) -> [VSCP_ComboKeyEn_flg]
  Signal Status Detection/2(VSCP_ComboKeyEnCMD_flg) -> [VSCP_ComboKeyEnCMD_flg]
  VINP_SWC2LScrollDownSta_flg/1 -> [VINP_SWCSetdownSta_flg]
  [VINP_SWCResUpSta_flg] -> Signal Status Detection/4(VINP_SWCResUpSta_flg)
  VINP_SWC2RegenDown_flg/1 -> [VINP_SWCRegenDown_flg]
  Signal Status Detection/4(VSCP_ComboKeyEnter_flg) -> [VSCP_ComboKeyEnter_flg]
  [VINP_SWCUpSta_flg] -> Signal Status Detection/6(VINP_SWCUpSta_flg)
  [VINP_PwrSta_enum] -> Operation Condition/1(VINP_PwrSta_enum)
  [VINP_SWCDownSta_flg] -> Signal Status Detection/7(VINP_SWCDownSta_flg)
  [VSCP_ComboKeyEnCMD_flg] -> Operation Condition/3(VSCP_ComboKeyEnCMD_flg)
  [VINP_SWCRegenUp_flg] -> Signal Status Detection/3(VINP_SWCRegenUp_flg)
  VINP_SWC2RegenUp_flg/1 -> [VINP_SWCRegenUp_flg]
  [VINP_SWCSetdownSta_flg] -> Signal Status Detection/5(VINP_SWCSetdownSta_flg)
  [VINP_SWCRegenDown_flg] -> Signal Status Detection/2(VINP_SWCRegenDown_flg)
  Operation Condition/1(VSCP_ComboKeyPreEn_flg) -> [VSCP_ComboKeyPreEn_flg]
  [TASK_TIME_10_MS] -> Signal Status Detection/1(TASK_TIME_10_MS)
  [VSCP_StreetFightMode_flg] -> VTQD_StreetFightMode_flg/1
  Signal Status Detection/1(VSCP_ComboKey_enum) -> [VSCP_ComboKey_enum]
  [VSCP_ComboKeyPreEn_flg] -> Signal Status Detection/9(VSCP_ComboKeyPreEn_flg)
